simulink model "MuscleSpindle"  (Simulink 7.9)
settings: Solver=ode3  StartTime=0.0  StopTime=inf  FixedStep=1e-3  MinStep=1e-12  RelTol=1e-4
settings Model: MinMaxOverflowLogging=ForceOff  Creator=oli  LastModifiedBy=oli  BufferReuse=off
settings DataIOCC: SaveOutput=off  SaveTime=off
settings OptimizationCC: BlockReduction=off  InlineParams=on  BufferReuse=off
settings DebuggingCC: AlgebraicLoopMsg=none  SolverPrmCheckMsg=none  UnconnectedInputMsg=none  UnconnectedOutputMsg=none  UnconnectedLineMsg=none

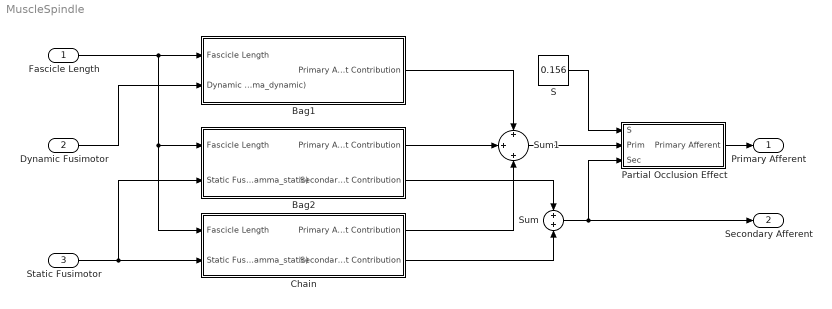
== system MuscleSpindle ==
  Fascicle Length : Inport
  Dynamic Fusimotor : Inport  Port=2
  Static Fusimotor : Inport  Port=3
  Bag1 : Subsystem
  Bag2 : Subsystem
  Chain : Subsystem
  Partial Occlusion Effect : Subsystem
  S : Constant  Value=0.156
  Sum : Sum  Inputs=+|+
  Sum1 : Sum  Inputs=+|+|+
  Primary Afferent : Outport
  Secondary Afferent : Outport  Port=2
  wires:
  Fascicle Length/1 -> Bag2/1(Fascicle Length), Chain/1(Fascicle Length), Bag1/1(Fascicle Length)
  Dynamic Fusimotor/1 -> Bag1/2(Dynamic Fusimotor (Gamma_dynamic))
  Static Fusimotor/1 -> Bag2/2(Static Fusimotor (Gamma_static)), Chain/2(Static Fusimotor (Gamma_static))
  Sum/1 -> Secondary Afferent/1, Partial Occlusion Effect/3(Sec)
  Partial Occlusion Effect/1(Primary Afferent) -> Primary Afferent/1
  Bag2/2(Secondary Afferent Contribution) -> Sum/1
  Bag1/1(Primary Afferent Contribution) -> Sum1/1
  Bag2/1(Primary Afferent Contribution) -> Sum1/2
  Chain/1(Primary Afferent Contribution) -> Sum1/3
  Chain/2(Secondary Afferent Contribution) -> Sum/2
  Sum1/1 -> Partial Occlusion Effect/2(Prim)
  S/1 -> Partial Occlusion Effect/1(S)

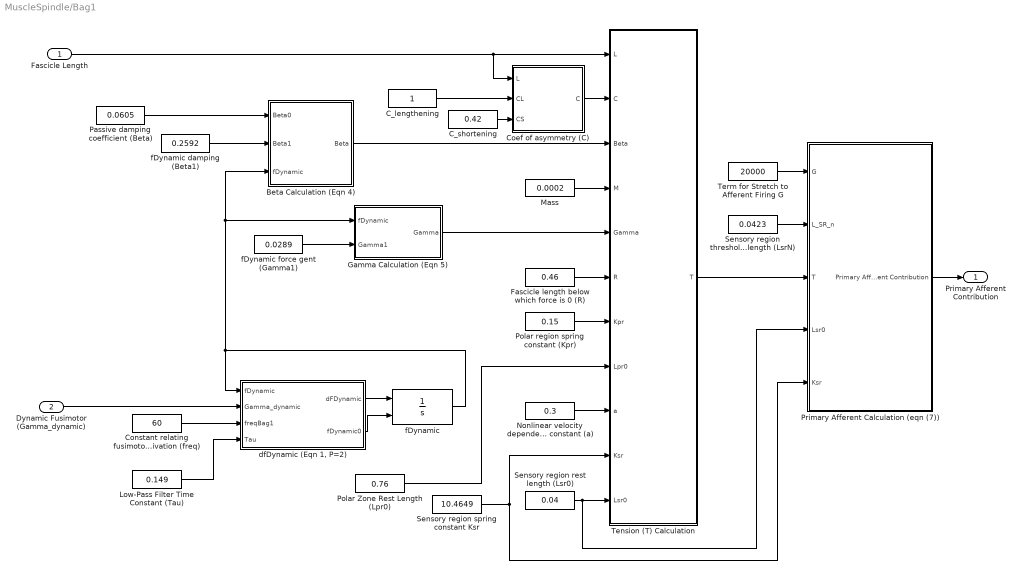
== system MuscleSpindle/Bag1 ==
  Fascicle Length : Inport
  Dynamic Fusimotor (Gamma_dynamic) : Inport  Port=2
  Beta Calculation (Eqn 4) : Subsystem
  C_lengthening : Constant
  C_shortening : Constant  Value=0.42
  Coef of asymmetry (C) : Subsystem
  Constant relating fusimotor frequency to activation (freq) : Constant  Value=60
  Fascicle length below which force is 0 (R) : Constant  Value=0.46
  Gamma Calculation (Eqn 5) : Subsystem
  Low-Pass Filter Time Constant (Tau) : Constant  Value=0.149
  Mass : Constant  Value=0.0002
  Nonlinear velocity dependence power constant (a) : Constant  Value=0.3
  Passive damping coefficient (Beta) : Constant  Value=0.0605
  Polar Zone Rest Length (Lpr0) : Constant  Value=0.76
  Polar region spring constant (Kpr) : Constant  Value=0.15
  Primary Afferent Calculation (eqn (7)) : Subsystem
  Sensory region rest length (Lsr0) : Constant  Value=0.04
  Sensory region spring constant Ksr : Constant  Value=10.4649
  Sensory region threshold length (LsrN) : Constant  Value=0.0423
  "Tension (T) Calculation " : Subsystem
  Term for Stretch to Afferent Firing G : Constant  Value=20000
  "dfDynamic (Eqn 1, P=2)" : Subsystem
  fDynamic : Integrator  InitialConditionSource=external
  fDynamic damping (Beta1) : Constant  Value=0.2592
  fDynamic force gent (Gamma1) : Constant  Value=0.0289
  Primary Afferent Contribution : Outport
  wires:
  Polar Zone Rest Length (Lpr0)/1 -> "Tension (T) Calculation "/8(Lpr0)
  fDynamic/1 -> Beta Calculation (Eqn 4)/3(fDynamic), Gamma Calculation (Eqn 5)/1(fDynamic), "dfDynamic (Eqn 1, P=2)"/1(fDynamic)
  "dfDynamic (Eqn 1, P=2)"/1(dFDynamic) -> fDynamic/1
  Dynamic Fusimotor (Gamma_dynamic)/1 -> "dfDynamic (Eqn 1, P=2)"/2(Gamma_dynamic)
  Low-Pass Filter Time Constant (Tau)/1 -> "dfDynamic (Eqn 1, P=2)"/4(Tau)
  Constant relating fusimotor frequency to activation (freq)/1 -> "dfDynamic (Eqn 1, P=2)"/3(freqBag1)
  Primary Afferent Calculation (eqn (7))/1(Primary Afferent Contribution) -> Primary Afferent Contribution/1
  "Tension (T) Calculation "/1(T) -> Primary Afferent Calculation (eqn (7))/3(T)
  Term for Stretch to Afferent Firing G/1 -> Primary Afferent Calculation (eqn (7))/1(G)
  Sensory region spring constant Ksr/1 -> Primary Afferent Calculation (eqn (7))/5(Ksr), "Tension (T) Calculation "/10(Ksr)
  Sensory region rest length (Lsr0)/1 -> Primary Afferent Calculation (eqn (7))/4(Lsr0), "Tension (T) Calculation "/11(Lsr0)
  Sensory region threshold length (LsrN)/1 -> Primary Afferent Calculation (eqn (7))/2(L_SR_n)
  Passive damping coefficient (Beta)/1 -> Beta Calculation (Eqn 4)/1(Beta0)
  Beta Calculation (Eqn 4)/1(Beta) -> "Tension (T) Calculation "/3(Beta)
  fDynamic damping (Beta1)/1 -> Beta Calculation (Eqn 4)/2(Beta1)
  Mass/1 -> "Tension (T) Calculation "/4(M)
  fDynamic force gent (Gamma1)/1 -> Gamma Calculation (Eqn 5)/2(Gamma1)
  Fascicle Length/1 -> "Tension (T) Calculation "/1(L), Coef of asymmetry (C)/1(L)
  Fascicle length below which force is 0 (R)/1 -> "Tension (T) Calculation "/6(R)
  Gamma Calculation (Eqn 5)/1(Gamma) -> "Tension (T) Calculation "/5(Gamma)
  C_lengthening/1 -> Coef of asymmetry (C)/2(CL)
  C_shortening/1 -> Coef of asymmetry (C)/3(CS)
  Coef of asymmetry (C)/1(C) -> "Tension (T) Calculation "/2(C)
  Nonlinear velocity dependence power constant (a)/1 -> "Tension (T) Calculation "/9(a)
  Polar region spring constant (Kpr)/1 -> "Tension (T) Calculation "/7(Kpr)
  "dfDynamic (Eqn 1, P=2)"/2(fDynamic0) -> fDynamic/2

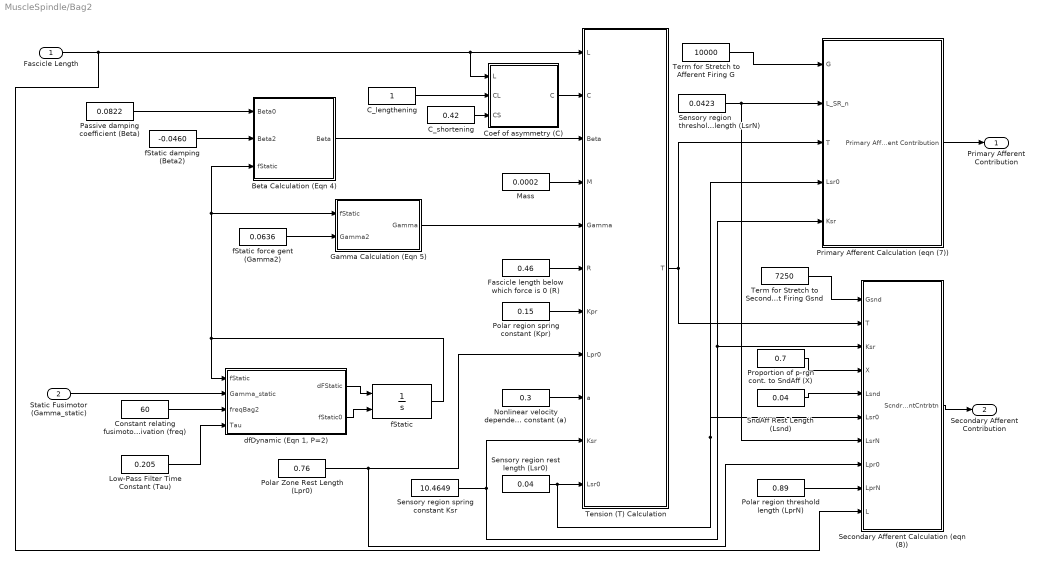
== system MuscleSpindle/Bag2 ==
  Fascicle Length : Inport
  Static Fusimotor (Gamma_static) : Inport  Port=2
  Beta Calculation (Eqn 4) : Subsystem
  C_lengthening : Constant
  C_shortening : Constant  Value=0.42
  Coef of asymmetry (C) : Subsystem
  Constant relating fusimotor frequency to activation (freq) : Constant  Value=60
  Fascicle length below which force is 0 (R) : Constant  Value=0.46
  Gamma Calculation (Eqn 5) : Subsystem
  Low-Pass Filter Time Constant (Tau) : Constant  Value=0.205
  Mass : Constant  Value=0.0002
  Nonlinear velocity dependence power constant (a) : Constant  Value=0.3
  Passive damping coefficient (Beta) : Constant  Value=0.0822
  Polar Zone Rest Length (Lpr0) : Constant  Value=0.76
  Polar region spring constant (Kpr) : Constant  Value=0.15
  Polar region threshold length (LprN) : Constant  Value=0.89
  Primary Afferent Calculation (eqn (7)) : Subsystem
  Proportion of p-rgn cont. to SndAff (X) : Constant  Value=0.7
  Secondary Afferent Calculation (eqn (8)) : MATLAB Function  TreatAsAtomicUnit=on
  Sensory region rest length (Lsr0) : Constant  Value=0.04
  Sensory region spring constant Ksr : Constant  Value=10.4649
  Sensory region threshold length (LsrN) : Constant  Value=0.0423
  SndAff Rest Length (Lsnd) : Constant  Value=0.04
  "Tension (T) Calculation " : Subsystem
  Term for Stretch to Afferent Firing G : Constant  Value=10000
  Term for Stretch to Secondary Afferent Firing Gsnd : Constant  Value=7250
  "dfDynamic (Eqn 1, P=2)" : Subsystem
  fStatic : Integrator  InitialConditionSource=external
  fStatic damping (Beta2) : Constant  Value=-0.0460
  fStatic force gent (Gamma2) : Constant  Value=0.0636
  Primary Afferent Contribution : Outport
  Secondary Afferent Contribution : Outport  Port=2
  wires:
  Polar Zone Rest Length (Lpr0)/1 -> "Tension (T) Calculation "/8(Lpr0), Secondary Afferent Calculation (eqn (8))/8(Lpr0)
  fStatic/1 -> Beta Calculation (Eqn 4)/3(fStatic), Gamma Calculation (Eqn 5)/1(fStatic), "dfDynamic (Eqn 1, P=2)"/1(fStatic)
  "dfDynamic (Eqn 1, P=2)"/1(dFStatic) -> fStatic/1
  Static Fusimotor (Gamma_static)/1 -> "dfDynamic (Eqn 1, P=2)"/2(Gamma_static)
  Low-Pass Filter Time Constant (Tau)/1 -> "dfDynamic (Eqn 1, P=2)"/4(Tau)
  Constant relating fusimotor frequency to activation (freq)/1 -> "dfDynamic (Eqn 1, P=2)"/3(freqBag2)
  Primary Afferent Calculation (eqn (7))/1(Primary Afferent Contribution) -> Primary Afferent Contribution/1
  "Tension (T) Calculation "/1(T) -> Primary Afferent Calculation (eqn (7))/3(T), Secondary Afferent Calculation (eqn (8))/2(T)
  Term for Stretch to Afferent Firing G/1 -> Primary Afferent Calculation (eqn (7))/1(G)
  Sensory region spring constant Ksr/1 -> "Tension (T) Calculation "/10(Ksr), Primary Afferent Calculation (eqn (7))/5(Ksr), Secondary Afferent Calculation (eqn (8))/3(Ksr)
  Sensory region rest length (Lsr0)/1 -> "Tension (T) Calculation "/11(Lsr0), Primary Afferent Calculation (eqn (7))/4(Lsr0), Secondary Afferent Calculation (eqn (8))/6(Lsr0)
  Sensory region threshold length (LsrN)/1 -> Primary Afferent Calculation (eqn (7))/2(L_SR_n), Secondary Afferent Calculation (eqn (8))/7(LsrN)
  Passive damping coefficient (Beta)/1 -> Beta Calculation (Eqn 4)/1(Beta0)
  Beta Calculation (Eqn 4)/1(Beta) -> "Tension (T) Calculation "/3(Beta)
  fStatic damping (Beta2)/1 -> Beta Calculation (Eqn 4)/2(Beta2)
  Mass/1 -> "Tension (T) Calculation "/4(M)
  fStatic force gent (Gamma2)/1 -> Gamma Calculation (Eqn 5)/2(Gamma2)
  Fascicle Length/1 -> "Tension (T) Calculation "/1(L), Coef of asymmetry (C)/1(L), Secondary Afferent Calculation (eqn (8))/10(L)
  Fascicle length below which force is 0 (R)/1 -> "Tension (T) Calculation "/6(R)
  Gamma Calculation (Eqn 5)/1(Gamma) -> "Tension (T) Calculation "/5(Gamma)
  C_lengthening/1 -> Coef of asymmetry (C)/2(CL)
  C_shortening/1 -> Coef of asymmetry (C)/3(CS)
  Coef of asymmetry (C)/1(C) -> "Tension (T) Calculation "/2(C)
  Nonlinear velocity dependence power constant (a)/1 -> "Tension (T) Calculation "/9(a)
  Polar region spring constant (Kpr)/1 -> "Tension (T) Calculation "/7(Kpr)
  Secondary Afferent Calculation (eqn (8))/1(ScndryAffrntCntrbtn) -> Secondary Afferent Contribution/1
  Term for Stretch to Secondary Afferent Firing Gsnd/1 -> Secondary Afferent Calculation (eqn (8))/1(Gsnd)
  Proportion of p-rgn cont. to SndAff (X)/1 -> Secondary Afferent Calculation (eqn (8))/4(X)
  SndAff Rest Length (Lsnd)/1 -> Secondary Afferent Calculation (eqn (8))/5(Lsnd)
  Polar region threshold length (LprN)/1 -> Secondary Afferent Calculation (eqn (8))/9(LprN)
  "dfDynamic (Eqn 1, P=2)"/2(fStatic0) -> fStatic/2

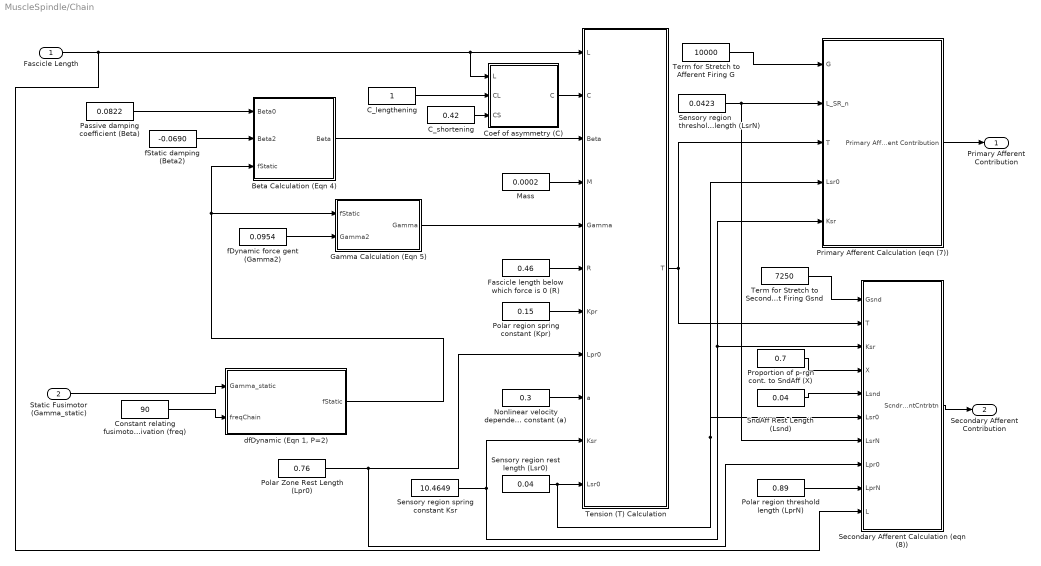
== system MuscleSpindle/Chain ==
  Fascicle Length : Inport
  Static Fusimotor (Gamma_static) : Inport  Port=2
  Beta Calculation (Eqn 4) : Subsystem
  C_lengthening : Constant
  C_shortening : Constant  Value=0.42
  Coef of asymmetry (C) : Subsystem
  Constant relating fusimotor frequency to activation (freq) : Constant  Value=90
  Fascicle length below which force is 0 (R) : Constant  Value=0.46
  Gamma Calculation (Eqn 5) : Subsystem
  Mass : Constant  Value=0.0002
  Nonlinear velocity dependence power constant (a) : Constant  Value=0.3
  Passive damping coefficient (Beta) : Constant  Value=0.0822
  Polar Zone Rest Length (Lpr0) : Constant  Value=0.76
  Polar region spring constant (Kpr) : Constant  Value=0.15
  Polar region threshold length (LprN) : Constant  Value=0.89
  Primary Afferent Calculation (eqn (7)) : Subsystem
  Proportion of p-rgn cont. to SndAff (X) : Constant  Value=0.7
  Secondary Afferent Calculation (eqn (8)) : MATLAB Function  TreatAsAtomicUnit=on
  Sensory region rest length (Lsr0) : Constant  Value=0.04
  Sensory region spring constant Ksr : Constant  Value=10.4649
  Sensory region threshold length (LsrN) : Constant  Value=0.0423
  SndAff Rest Length (Lsnd) : Constant  Value=0.04
  "Tension (T) Calculation " : Subsystem
  Term for Stretch to Afferent Firing G : Constant  Value=10000
  Term for Stretch to Secondary Afferent Firing Gsnd : Constant  Value=7250
  "dfDynamic (Eqn 1, P=2)" : Subsystem
  fDynamic force gent (Gamma2) : Constant  Value=0.0954
  fStatic damping (Beta2) : Constant  Value=-0.0690
  Primary Afferent Contribution : Outport
  Secondary Afferent Contribution : Outport  Port=2
  wires:
  Polar Zone Rest Length (Lpr0)/1 -> "Tension (T) Calculation "/8(Lpr0), Secondary Afferent Calculation (eqn (8))/8(Lpr0)
  "dfDynamic (Eqn 1, P=2)"/1(fStatic) -> Beta Calculation (Eqn 4)/3(fStatic), Gamma Calculation (Eqn 5)/1(fStatic)
  Static Fusimotor (Gamma_static)/1 -> "dfDynamic (Eqn 1, P=2)"/1(Gamma_static)
  Constant relating fusimotor frequency to activation (freq)/1 -> "dfDynamic (Eqn 1, P=2)"/2(freqChain)
  Primary Afferent Calculation (eqn (7))/1(Primary Afferent Contribution) -> Primary Afferent Contribution/1
  "Tension (T) Calculation "/1(T) -> Primary Afferent Calculation (eqn (7))/3(T), Secondary Afferent Calculation (eqn (8))/2(T)
  Term for Stretch to Afferent Firing G/1 -> Primary Afferent Calculation (eqn (7))/1(G)
  Sensory region spring constant Ksr/1 -> "Tension (T) Calculation "/10(Ksr), Primary Afferent Calculation (eqn (7))/5(Ksr), Secondary Afferent Calculation (eqn (8))/3(Ksr)
  Sensory region rest length (Lsr0)/1 -> "Tension (T) Calculation "/11(Lsr0), Primary Afferent Calculation (eqn (7))/4(Lsr0), Secondary Afferent Calculation (eqn (8))/6(Lsr0)
  Sensory region threshold length (LsrN)/1 -> Primary Afferent Calculation (eqn (7))/2(L_SR_n), Secondary Afferent Calculation (eqn (8))/7(LsrN)
  Passive damping coefficient (Beta)/1 -> Beta Calculation (Eqn 4)/1(Beta0)
  Beta Calculation (Eqn 4)/1(Beta) -> "Tension (T) Calculation "/3(Beta)
  fStatic damping (Beta2)/1 -> Beta Calculation (Eqn 4)/2(Beta2)
  Mass/1 -> "Tension (T) Calculation "/4(M)
  fDynamic force gent (Gamma2)/1 -> Gamma Calculation (Eqn 5)/2(Gamma2)
  Fascicle Length/1 -> "Tension (T) Calculation "/1(L), Coef of asymmetry (C)/1(L), Secondary Afferent Calculation (eqn (8))/10(L)
  Fascicle length below which force is 0 (R)/1 -> "Tension (T) Calculation "/6(R)
  Gamma Calculation (Eqn 5)/1(Gamma) -> "Tension (T) Calculation "/5(Gamma)
  C_lengthening/1 -> Coef of asymmetry (C)/2(CL)
  C_shortening/1 -> Coef of asymmetry (C)/3(CS)
  Coef of asymmetry (C)/1(C) -> "Tension (T) Calculation "/2(C)
  Nonlinear velocity dependence power constant (a)/1 -> "Tension (T) Calculation "/9(a)
  Polar region spring constant (Kpr)/1 -> "Tension (T) Calculation "/7(Kpr)
  Secondary Afferent Calculation (eqn (8))/1(ScndryAffrntCntrbtn) -> Secondary Afferent Contribution/1
  Term for Stretch to Secondary Afferent Firing Gsnd/1 -> Secondary Afferent Calculation (eqn (8))/1(Gsnd)
  Proportion of p-rgn cont. to SndAff (X)/1 -> Secondary Afferent Calculation (eqn (8))/4(X)
  SndAff Rest Length (Lsnd)/1 -> Secondary Afferent Calculation (eqn (8))/5(Lsnd)
  Polar region threshold length (LprN)/1 -> Secondary Afferent Calculation (eqn (8))/9(LprN)

== system MuscleSpindle/Partial Occlusion Effect ==
  S : Inport
  Prim : Inport  Port=2
  Sec : Inport  Port=3
  Max : MinMax  Function=max  Inputs=2
  Min : MinMax  Inputs=2
  Product : Product  RndMeth=Zero
  Sum : Sum  Inputs=|++
  Primary Afferent : Outport
  wires:
  Prim/1 -> Max/1, Min/1
  Sec/1 -> Max/2, Min/2
  Sum/1 -> Primary Afferent/1
  S/1 -> Product/1
  Min/1 -> Product/2
  Product/1 -> Sum/1
  Max/1 -> Sum/2

== system MuscleSpindle/Bag1/Beta Calculation (Eqn 4) ==
  Beta0 : Inport
  Beta1 : Inport  Port=2
  fDynamic : Inport  Port=3
  Add : Sum
  Product : Product  RndMeth=Zero
  Beta : Outport
  wires:
  Beta1/1 -> Product/1
  fDynamic/1 -> Product/2
  Add/1 -> Beta/1
  Beta0/1 -> Add/1
  Product/1 -> Add/2

== system MuscleSpindle/Bag1/Coef of asymmetry (C) ==
  L : Inport
  CL : Inport  Port=2
  CS : Inport  Port=3
  Model : ModelReference  ModelNameDialog=ContinuousDetectIncrease  SimulationMode=Normal  ModelReferenceVersion=1.21  CopyOfModelName=ContinuousDetectIncrease  DefaultDataLogging=on
  Rate Transition : RateTransition
  Rate Transition1 : RateTransition
  Switch : Switch
  C : Outport
  wires:
  CL/1 -> Switch/1
  CS/1 -> Switch/3
  Model/1 -> Switch/2
  L/1 -> Rate Transition/1
  Rate Transition/1 -> Model/1
  Switch/1 -> Rate Transition1/1
  Rate Transition1/1 -> C/1

== system MuscleSpindle/Bag1/Gamma Calculation (Eqn 5) ==
  fDynamic : Inport
  Gamma1 : Inport  Port=2
  Product : Product  RndMeth=Zero
  Gamma : Outport
  wires:
  Product/1 -> Gamma/1
  Gamma1/1 -> Product/1
  fDynamic/1 -> Product/2

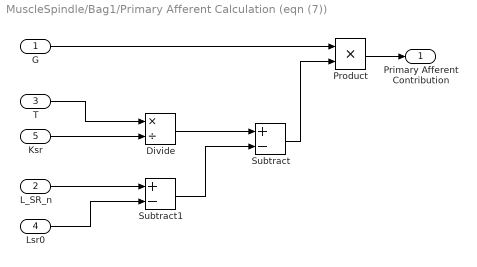
== system MuscleSpindle/Bag1/Primary Afferent Calculation (eqn (7)) ==
  G : Inport
  L_SR_n : Inport  Port=2
  T : Inport  Port=3
  Lsr0 : Inport  Port=4
  Ksr : Inport  Port=5
  Divide : Product  Inputs=*/
  Product : Product  RndMeth=Zero
  Subtract : Sum  Inputs=+-
  Subtract1 : Sum  Inputs=+-
  Primary Afferent Contribution : Outport
  wires:
  G/1 -> Product/1
  Product/1 -> Primary Afferent Contribution/1
  Subtract/1 -> Product/2
  T/1 -> Divide/1
  Ksr/1 -> Divide/2
  Divide/1 -> Subtract/1
  L_SR_n/1 -> Subtract1/1
  Lsr0/1 -> Subtract1/2
  Subtract1/1 -> Subtract/2

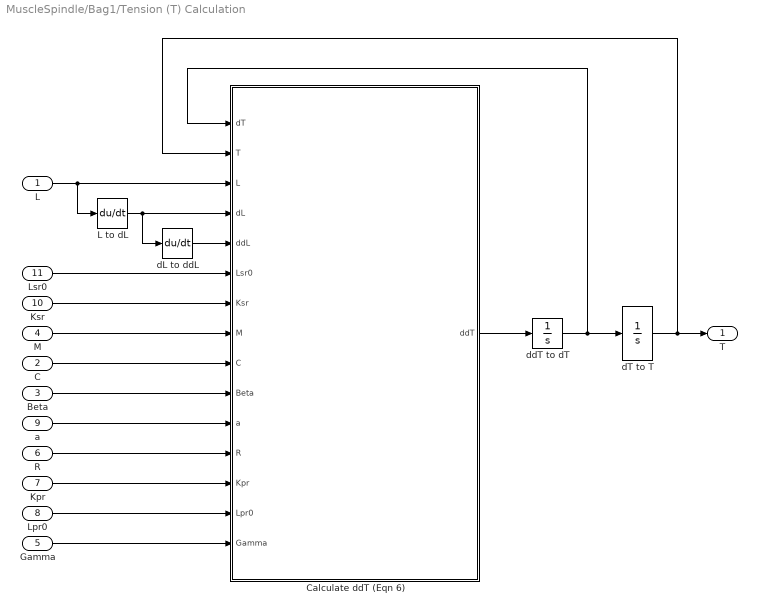
== system MuscleSpindle/Bag1/Tension (T) Calculation  ==
  L : Inport
  C : Inport  Port=2
  Beta : Inport  Port=3
  M : Inport  Port=4
  Gamma : Inport  Port=5
  R : Inport  Port=6
  Kpr : Inport  Port=7
  Lpr0 : Inport  Port=8
  a : Inport  Port=9
  Ksr : Inport  Port=10
  Lsr0 : Inport  Port=11
  Calculate ddT (Eqn 6) : MATLAB Function  TreatAsAtomicUnit=on
  L to dL : Derivative  CoefficientInTFapproximation=Inf
  dL to ddL : Derivative  CoefficientInTFapproximation=Inf
  dT to T : Integrator
  ddT to dT : Integrator
  T : Outport
  wires:
  L/1 -> L to dL/1, Calculate ddT (Eqn 6)/3(L)
  Lsr0/1 -> Calculate ddT (Eqn 6)/6(Lsr0)
  Gamma/1 -> Calculate ddT (Eqn 6)/15(Gamma)
  Kpr/1 -> Calculate ddT (Eqn 6)/13(Kpr)
  a/1 -> Calculate ddT (Eqn 6)/11(a)
  C/1 -> Calculate ddT (Eqn 6)/9(C)
  Lpr0/1 -> Calculate ddT (Eqn 6)/14(Lpr0)
  Beta/1 -> Calculate ddT (Eqn 6)/10(Beta)
  Ksr/1 -> Calculate ddT (Eqn 6)/7(Ksr)
  M/1 -> Calculate ddT (Eqn 6)/8(M)
  R/1 -> Calculate ddT (Eqn 6)/12(R)
  Calculate ddT (Eqn 6)/1(ddT) -> ddT to dT/1
  ddT to dT/1 -> dT to T/1, Calculate ddT (Eqn 6)/1(dT)
  dT to T/1 -> T/1, Calculate ddT (Eqn 6)/2(T)
  L to dL/1 -> dL to ddL/1, Calculate ddT (Eqn 6)/4(dL)
  dL to ddL/1 -> Calculate ddT (Eqn 6)/5(ddL)

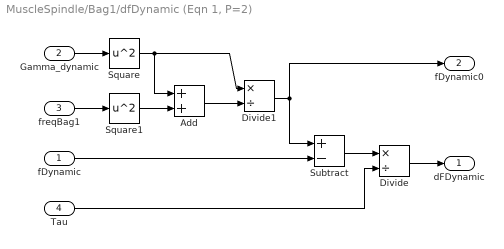
== system MuscleSpindle/Bag1/dfDynamic (Eqn 1, P=2) ==
  fDynamic : Inport
  Gamma_dynamic : Inport  Port=2
  freqBag1 : Inport  Port=3
  Tau : Inport  Port=4
  Add : Sum
  Divide : Product  Inputs=*/
  Divide1 : Product  Inputs=*/
  Square : Math  Operator=square  SaturateOnIntegerOverflow=on
  Square1 : Math  Operator=square  SaturateOnIntegerOverflow=on
  Subtract : Sum  Inputs=+-
  dFDynamic : Outport
  fDynamic0 : Outport  Port=2
  wires:
  Divide/1 -> dFDynamic/1
  Tau/1 -> Divide/2
  Subtract/1 -> Divide/1
  fDynamic/1 -> Subtract/2
  Divide1/1 -> Subtract/1, fDynamic0/1
  Add/1 -> Divide1/2
  Gamma_dynamic/1 -> Square/1
  Square/1 -> Divide1/1, Add/1
  freqBag1/1 -> Square1/1
  Square1/1 -> Add/2

== system MuscleSpindle/Bag2/Beta Calculation (Eqn 4) ==
  Beta0 : Inport
  Beta2 : Inport  Port=2
  fStatic : Inport  Port=3
  Add : Sum
  Product : Product  RndMeth=Zero
  Beta : Outport
  wires:
  Beta2/1 -> Product/1
  fStatic/1 -> Product/2
  Add/1 -> Beta/1
  Beta0/1 -> Add/1
  Product/1 -> Add/2

== system MuscleSpindle/Bag2/Coef of asymmetry (C) ==
  L : Inport
  CL : Inport  Port=2
  CS : Inport  Port=3
  Model : ModelReference  ModelNameDialog=ContinuousDetectIncrease  SimulationMode=Normal  ModelReferenceVersion=1.21  CopyOfModelName=ContinuousDetectIncrease  DefaultDataLogging=on
  Rate Transition : RateTransition
  Rate Transition1 : RateTransition
  Switch : Switch
  C : Outport
  wires:
  CL/1 -> Switch/1
  CS/1 -> Switch/3
  Model/1 -> Switch/2
  L/1 -> Rate Transition/1
  Rate Transition/1 -> Model/1
  Switch/1 -> Rate Transition1/1
  Rate Transition1/1 -> C/1

== system MuscleSpindle/Bag2/Gamma Calculation (Eqn 5) ==
  fStatic : Inport
  Gamma2 : Inport  Port=2
  Product : Product  RndMeth=Zero
  Gamma : Outport
  wires:
  Product/1 -> Gamma/1
  Gamma2/1 -> Product/1
  fStatic/1 -> Product/2

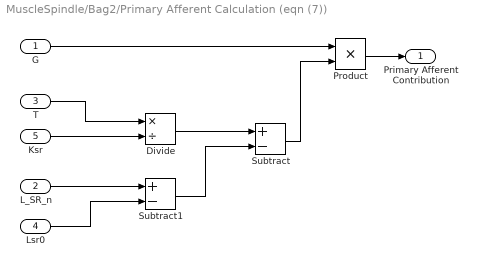
== system MuscleSpindle/Bag2/Primary Afferent Calculation (eqn (7)) ==
  G : Inport
  L_SR_n : Inport  Port=2
  T : Inport  Port=3
  Lsr0 : Inport  Port=4
  Ksr : Inport  Port=5
  Divide : Product  Inputs=*/
  Product : Product  RndMeth=Zero
  Subtract : Sum  Inputs=+-
  Subtract1 : Sum  Inputs=+-
  Primary Afferent Contribution : Outport
  wires:
  G/1 -> Product/1
  Product/1 -> Primary Afferent Contribution/1
  Subtract/1 -> Product/2
  T/1 -> Divide/1
  Ksr/1 -> Divide/2
  Divide/1 -> Subtract/1
  L_SR_n/1 -> Subtract1/1
  Lsr0/1 -> Subtract1/2
  Subtract1/1 -> Subtract/2

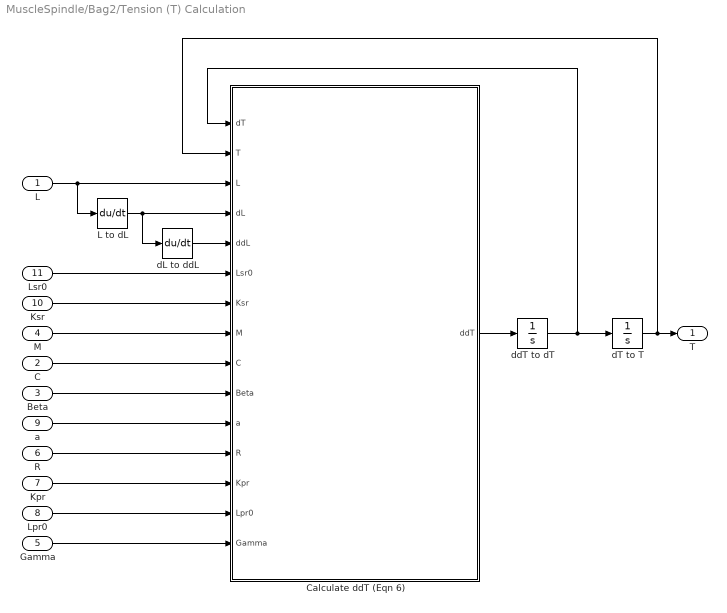
== system MuscleSpindle/Bag2/Tension (T) Calculation  ==
  L : Inport
  C : Inport  Port=2
  Beta : Inport  Port=3
  M : Inport  Port=4
  Gamma : Inport  Port=5
  R : Inport  Port=6
  Kpr : Inport  Port=7
  Lpr0 : Inport  Port=8
  a : Inport  Port=9
  Ksr : Inport  Port=10
  Lsr0 : Inport  Port=11
  Calculate ddT (Eqn 6) : MATLAB Function  TreatAsAtomicUnit=on
  L to dL : Derivative  CoefficientInTFapproximation=Inf
  dL to ddL : Derivative  CoefficientInTFapproximation=Inf
  dT to T : Integrator
  ddT to dT : Integrator
  T : Outport
  wires:
  L/1 -> Calculate ddT (Eqn 6)/3(L), L to dL/1
  Lsr0/1 -> Calculate ddT (Eqn 6)/6(Lsr0)
  Gamma/1 -> Calculate ddT (Eqn 6)/15(Gamma)
  Kpr/1 -> Calculate ddT (Eqn 6)/13(Kpr)
  a/1 -> Calculate ddT (Eqn 6)/11(a)
  C/1 -> Calculate ddT (Eqn 6)/9(C)
  Lpr0/1 -> Calculate ddT (Eqn 6)/14(Lpr0)
  Beta/1 -> Calculate ddT (Eqn 6)/10(Beta)
  Ksr/1 -> Calculate ddT (Eqn 6)/7(Ksr)
  M/1 -> Calculate ddT (Eqn 6)/8(M)
  R/1 -> Calculate ddT (Eqn 6)/12(R)
  Calculate ddT (Eqn 6)/1(ddT) -> ddT to dT/1
  ddT to dT/1 -> dT to T/1, Calculate ddT (Eqn 6)/1(dT)
  dT to T/1 -> T/1, Calculate ddT (Eqn 6)/2(T)
  L to dL/1 -> Calculate ddT (Eqn 6)/4(dL), dL to ddL/1
  dL to ddL/1 -> Calculate ddT (Eqn 6)/5(ddL)

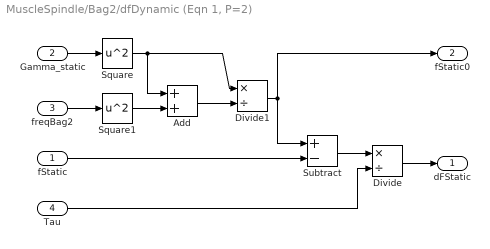
== system MuscleSpindle/Bag2/dfDynamic (Eqn 1, P=2) ==
  fStatic : Inport
  Gamma_static : Inport  Port=2
  freqBag2 : Inport  Port=3
  Tau : Inport  Port=4
  Add : Sum
  Divide : Product  Inputs=*/
  Divide1 : Product  Inputs=*/
  Square : Math  Operator=square  SaturateOnIntegerOverflow=on
  Square1 : Math  Operator=square  SaturateOnIntegerOverflow=on
  Subtract : Sum  Inputs=+-
  dFStatic : Outport
  fStatic0 : Outport  Port=2
  wires:
  Divide/1 -> dFStatic/1
  Tau/1 -> Divide/2
  Subtract/1 -> Divide/1
  fStatic/1 -> Subtract/2
  Divide1/1 -> Subtract/1, fStatic0/1
  Add/1 -> Divide1/2
  Gamma_static/1 -> Square/1
  Square/1 -> Divide1/1, Add/1
  freqBag2/1 -> Square1/1
  Square1/1 -> Add/2

== system MuscleSpindle/Chain/Beta Calculation (Eqn 4) ==
  Beta0 : Inport
  Beta2 : Inport  Port=2
  fStatic : Inport  Port=3
  Add : Sum
  Product : Product  RndMeth=Zero
  Beta : Outport
  wires:
  Beta2/1 -> Product/1
  fStatic/1 -> Product/2
  Add/1 -> Beta/1
  Beta0/1 -> Add/1
  Product/1 -> Add/2

== system MuscleSpindle/Chain/Coef of asymmetry (C) ==
  L : Inport
  CL : Inport  Port=2
  CS : Inport  Port=3
  Model : ModelReference  ModelNameDialog=ContinuousDetectIncrease  SimulationMode=Normal  ModelReferenceVersion=1.21  CopyOfModelName=ContinuousDetectIncrease  DefaultDataLogging=on
  Rate Transition : RateTransition
  Rate Transition1 : RateTransition
  Switch : Switch
  C : Outport
  wires:
  CL/1 -> Switch/1
  CS/1 -> Switch/3
  Model/1 -> Switch/2
  L/1 -> Rate Transition/1
  Rate Transition/1 -> Model/1
  Switch/1 -> Rate Transition1/1
  Rate Transition1/1 -> C/1

== system MuscleSpindle/Chain/Gamma Calculation (Eqn 5) ==
  fStatic : Inport
  Gamma2 : Inport  Port=2
  Product : Product  RndMeth=Zero
  Gamma : Outport
  wires:
  Product/1 -> Gamma/1
  Gamma2/1 -> Product/1
  fStatic/1 -> Product/2

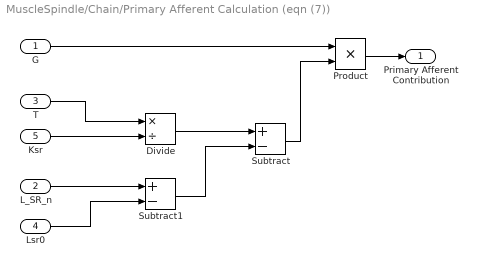
== system MuscleSpindle/Chain/Primary Afferent Calculation (eqn (7)) ==
  G : Inport
  L_SR_n : Inport  Port=2
  T : Inport  Port=3
  Lsr0 : Inport  Port=4
  Ksr : Inport  Port=5
  Divide : Product  Inputs=*/
  Product : Product  RndMeth=Zero
  Subtract : Sum  Inputs=+-
  Subtract1 : Sum  Inputs=+-
  Primary Afferent Contribution : Outport
  wires:
  G/1 -> Product/1
  Product/1 -> Primary Afferent Contribution/1
  Subtract/1 -> Product/2
  T/1 -> Divide/1
  Ksr/1 -> Divide/2
  Divide/1 -> Subtract/1
  L_SR_n/1 -> Subtract1/1
  Lsr0/1 -> Subtract1/2
  Subtract1/1 -> Subtract/2

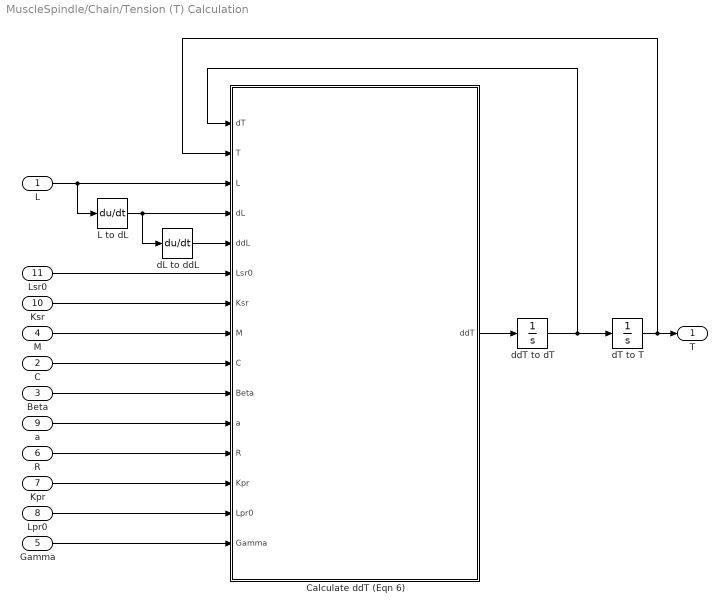
== system MuscleSpindle/Chain/Tension (T) Calculation  ==
  L : Inport
  C : Inport  Port=2
  Beta : Inport  Port=3
  M : Inport  Port=4
  Gamma : Inport  Port=5
  R : Inport  Port=6
  Kpr : Inport  Port=7
  Lpr0 : Inport  Port=8
  a : Inport  Port=9
  Ksr : Inport  Port=10
  Lsr0 : Inport  Port=11
  Calculate ddT (Eqn 6) : MATLAB Function  TreatAsAtomicUnit=on
  L to dL : Derivative  CoefficientInTFapproximation=Inf
  dL to ddL : Derivative  CoefficientInTFapproximation=Inf
  dT to T : Integrator
  ddT to dT : Integrator
  T : Outport
  wires:
  L/1 -> Calculate ddT (Eqn 6)/3(L), L to dL/1
  Lsr0/1 -> Calculate ddT (Eqn 6)/6(Lsr0)
  Gamma/1 -> Calculate ddT (Eqn 6)/15(Gamma)
  Kpr/1 -> Calculate ddT (Eqn 6)/13(Kpr)
  a/1 -> Calculate ddT (Eqn 6)/11(a)
  C/1 -> Calculate ddT (Eqn 6)/9(C)
  Lpr0/1 -> Calculate ddT (Eqn 6)/14(Lpr0)
  Beta/1 -> Calculate ddT (Eqn 6)/10(Beta)
  Ksr/1 -> Calculate ddT (Eqn 6)/7(Ksr)
  M/1 -> Calculate ddT (Eqn 6)/8(M)
  R/1 -> Calculate ddT (Eqn 6)/12(R)
  Calculate ddT (Eqn 6)/1(ddT) -> ddT to dT/1
  ddT to dT/1 -> dT to T/1, Calculate ddT (Eqn 6)/1(dT)
  dT to T/1 -> T/1, Calculate ddT (Eqn 6)/2(T)
  L to dL/1 -> Calculate ddT (Eqn 6)/4(dL), dL to ddL/1
  dL to ddL/1 -> Calculate ddT (Eqn 6)/5(ddL)

== system MuscleSpindle/Chain/dfDynamic (Eqn 1, P=2) ==
  Gamma_static : Inport
  freqChain : Inport  Port=2
  Add : Sum
  Divide1 : Product  Inputs=*/
  Square : Math  Operator=square  SaturateOnIntegerOverflow=on
  Square1 : Math  Operator=square  SaturateOnIntegerOverflow=on
  fStatic : Outport
  wires:
  Add/1 -> Divide1/2
  Gamma_static/1 -> Square/1
  Square/1 -> Divide1/1, Add/1
  freqChain/1 -> Square1/1
  Square1/1 -> Add/2
  Divide1/1 -> fStatic/1

== matlab function Bag2/Tension (T) Calculation /Calculate ddT (Eqn 6) ==
  data: dT input double; T input double; L input double; dL input double; ddL input double; Lsr0 input double; Ksr input double; ddT output double; M input double; C input double; Beta input double; a input double; R input double; Kpr input double; Lpr0 input double; Gamma input double
function ddT = Calculate_ddT(dT, T, L, dL, ddL, Lsr0, Ksr, M, C, Beta, a, R, Kpr, Lpr0, Gamma)

    LTerm = L - Lsr0 - T/Ksr;

    ddT = Ksr/M * (...
            C * Beta * sign(dL - dT/Ksr) * abs(dL - dT/Ksr)^a * (LTerm - R) ...
            + Kpr * (LTerm - Lpr0) ...
            + M * ddL ...
            + Gamma ...
            - T);
end

== matlab function Bag1/Tension (T) Calculation /Calculate ddT (Eqn 6) ==
  data: dT input double; T input double; L input double; dL input double; ddL input double; Lsr0 input double; Ksr input double; ddT output double; M input double; C input double; Beta input double; a input double; R input double; Kpr input double; Lpr0 input double; Gamma input double
function ddT  = Calculate_ddT(dT, T, L, dL, ddL, Lsr0, Ksr, M, C, Beta, a, R, Kpr, Lpr0, Gamma)

    LTerm = L - Lsr0 - T/Ksr;

    ddT = Ksr/M * (...
            C * Beta * sign(dL - dT/Ksr) * abs(dL - dT/Ksr)^a * (LTerm - R) ...
            + Kpr * (LTerm - Lpr0) ...
            + M * ddL ...
            + Gamma ...
            - T);
end

== matlab function Bag2/Secondary Afferent Calculation (eqn (8)) ==
  data: Gsnd input double; T input double; Ksr input double; X input double; ScndryAffrntCntrbtn output double; Lsnd input double; Lsr0 input double; LsrN input double; Lpr0 input double; LprN input double; L input double
function ScndryAffrntCntrbtn = SndAffContrib(Gsnd,T,Ksr,X,Lsnd,Lsr0,LsrN,Lpr0,LprN,L)
    
    term1 = Lsnd/Lsr0 * (T/Ksr - (LsrN - Lsr0)); %sensory stretch contribution
    
    term2 = Lsnd/Lpr0 * (L - T/Ksr - Lsr0 - LprN); %polar stretch contribution

    term = X * term1 + (1-X)*term2; %combine the two

    ScndryAffrntCntrbtn = Gsnd*term; %scale for firing rate
end

== matlab function Chain/Secondary Afferent Calculation (eqn (8)) ==
  data: Gsnd input double; T input double; Ksr input double; X input double; ScndryAffrntCntrbtn output double; Lsnd input double; Lsr0 input double; LsrN input double; Lpr0 input double; LprN input double; L input double
function ScndryAffrntCntrbtn = SndAffContrib(Gsnd,T,Ksr,X,Lsnd,Lsr0,LsrN,Lpr0,LprN,L)
    
    term1 = Lsnd/Lsr0 * (T/Ksr - (LsrN - Lsr0)); %sensory stretch contribution
    
    term2 = Lsnd/Lpr0 * (L - T/Ksr - Lsr0 - LprN); %polar stretch contribution

    term = X * term1 + (1-X)*term2; %combine the two

    ScndryAffrntCntrbtn = Gsnd*term; %scale for firing rate
end

== matlab function Chain/Tension (T) Calculation /Calculate ddT (Eqn 6) ==
  data: dT input double; T input double; L input double; dL input double; ddL input double; Lsr0 input double; Ksr input double; ddT output double; M input double; C input double; Beta input double; a input double; R input double; Kpr input double; Lpr0 input double; Gamma input double
function ddT = Calculate_ddT(dT, T, L, dL, ddL, Lsr0, Ksr, M, C, Beta, a, R, Kpr, Lpr0, Gamma)

    LTerm = L - Lsr0 - T/Ksr;

    ddT = Ksr/M * (...
            C * Beta * sign(dL - dT/Ksr) * abs(dL - dT/Ksr)^a * (LTerm - R) ...
            + Kpr * (LTerm - Lpr0) ...
            + M * ddL ...
            + Gamma ...
            - T);
end
